simulink model "parte2_ej2_GBClasico"  (R2019b)
settings: Solver=VariableStepAuto  StartTime=0.0  StopTime=10.0  RelTol=1e-3
values from neighbouring files (symbols this model uses):
  H = 3.5    [parte2_ej2_GeneradorBusInfinito.m]    (also in parte2_ej2_GeneradorBusInfinitoHP.m)
  KD = 10    [parte2_ej2_GeneradorBusInfinito.m]    (also in parte2_ej2_GeneradorBusInfinitoHP.m; parte2_eje2_HPModel.m = 0)
  KS = 0.757    [parte2_ej2_GeneradorBusInfinito.m]
  w0 = 2*pi*60    (= 376.991118431)    [parte2_ej2_GeneradorBusInfinito.m]    (also in parte2_ej2_GeneradorBusInfinitoHP.m)
settings Model: Creator=cjuar  LastModifiedBy=cjuar

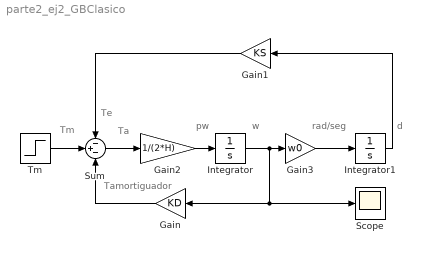
== system parte2_ej2_GBClasico ==
  note: d
  note: rad/seg
  note: w
  note: pw
  note: Ta
  note: Te
  note: Tamortiguador
  note: Tm
  Gain : Gain  Gain=KD
  Gain1 : Gain  Gain=KS
  Gain2 : Gain  Gain=1/(2*H)
  Gain3 : Gain  Gain=w0
  Integrator : Integrator
  Integrator1 : Integrator
  Scope : Scope
  Sum : Sum  Inputs=-+-
  Tm : Step  SampleTime=0
  wires:
  Tm/1 -> Sum/2
  Gain/1 -> Sum/3
  Gain1/1 -> Sum/1
  Sum/1 -> Gain2/1
  Gain2/1 -> Integrator/1
  Gain3/1 -> Integrator1/1
  Integrator1/1 -> Gain1/1
  Integrator/1 -> Gain3/1, Gain/1, Scope/1
